simulink model "RLC"  (Simulink 7.5)
settings: Solver=ode3  StartTime=0.0  StopTime=4  FixedStep=1/32000  RelTol=1e-3
InitFcn:
  | RLC_datastruct
StopFcn:
  | PostProcessing
values from neighbouring files (symbols this model uses):
  CValue = 0.00068    [RLC_datastruct.m]
  LValue = 0.001    [RLC_datastruct.m]
  RValue = 2    [RLC_datastruct.m]
libraries: dspsrcs4 x1
settings Model: Creator=Zsolt  LastModifiedBy=bapty

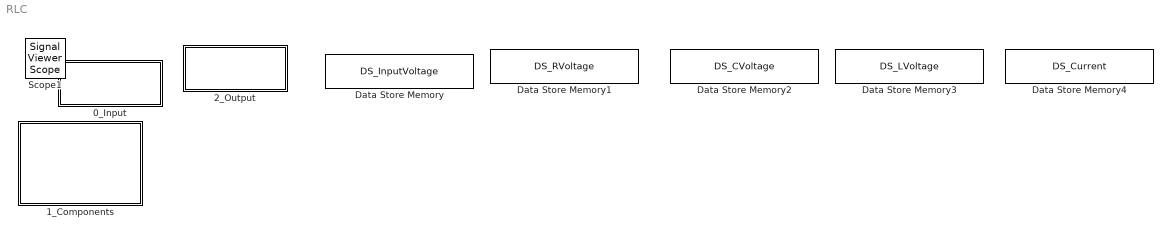
== system RLC ==
  0_Input : Subsystem
  1_Components : Subsystem
  2_Output : Subsystem
  Data Store Memory : DataStoreMemory  DataStoreName=DS_InputVoltage
  Data Store Memory1 : DataStoreMemory  DataStoreName=DS_RVoltage  ReadBeforeWriteMsg=warning  WriteAfterWriteMsg=warning  WriteAfterReadMsg=warning
  Data Store Memory2 : DataStoreMemory  DataStoreName=DS_CVoltage  ReadBeforeWriteMsg=warning  WriteAfterWriteMsg=warning  WriteAfterReadMsg=warning
  Data Store Memory3 : DataStoreMemory  DataStoreName=DS_LVoltage  ReadBeforeWriteMsg=warning  WriteAfterWriteMsg=warning  WriteAfterReadMsg=warning
  Data Store Memory4 : DataStoreMemory  DataStoreName=DS_Current  ReadBeforeWriteMsg=warning  WriteAfterWriteMsg=warning  WriteAfterReadMsg=warning
  Scope1 : SignalViewerScope  IOType=viewer  RefreshTime=0.035000

== system RLC/0_Input ==
  0_Chirp : dspsrcs4/Chirp  sweep=Linear  mode=Unidirectional  f0=1  f1=1000  t1=4  Tsweep=4  phase=0  Ts=1/32000  spf=1  datatype=Double
  1_Data Store Write : DataStoreWrite  DataStoreName=DS_InputVoltage  SampleTime=-1
  2_To Workspace : ToWorkspace  VariableName=InputVoltage  SampleTime=-1  SaveFormat=Structure With Time
  wires:
  0_Chirp/1 -> 1_Data Store Write/1, 2_To Workspace/1

== system RLC/1_Components ==
  RLC : Subsystem

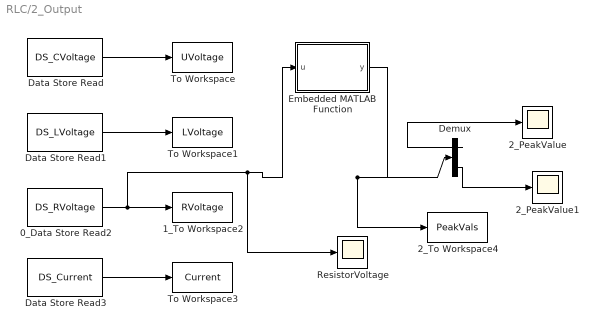
== system RLC/2_Output ==
  0_Data Store Read2 : DataStoreRead  DataStoreName=DS_RVoltage  SampleTime=-1
  1_To Workspace2 : ToWorkspace  VariableName=RVoltage  SampleTime=-1  SaveFormat=Structure With Time
  2_PeakValue : Scope
      settings: TimeRange=4  YMin=0  YMax=300  Decimation=10
  2_PeakValue1 : Scope
      settings: YMin=0  YMax=100  SaveName=ScopeData3  Decimation=10
  2_To Workspace4 : ToWorkspace  VariableName=PeakVals  SampleTime=-1  SaveFormat=Structure With Time
  Data Store Read : DataStoreRead  DataStoreName=DS_CVoltage  SampleTime=-1
  Data Store Read1 : DataStoreRead  DataStoreName=DS_LVoltage  SampleTime=-1
  Data Store Read3 : DataStoreRead  DataStoreName=DS_Current  SampleTime=-1
  Demux : Demux  Outputs=2
  Embedded MATLAB Function : Stateflow chart  TreatAsAtomicUnit=on
  ResistorVoltage : Scope
      settings: YMin=-1  YMax=1  SaveName=ScopeData2  Decimation=10
  To Workspace : ToWorkspace  VariableName=UVoltage  SampleTime=-1  SaveFormat=Structure With Time
  To Workspace1 : ToWorkspace  VariableName=LVoltage  SampleTime=-1  SaveFormat=Structure With Time
  To Workspace3 : ToWorkspace  VariableName=Current  SampleTime=-1  SaveFormat=Structure With Time
  wires:
  Data Store Read/1 -> To Workspace/1
  Data Store Read1/1 -> To Workspace1/1
  0_Data Store Read2/1 -> 1_To Workspace2/1, ResistorVoltage/1, Embedded MATLAB Function/1(u)
  Data Store Read3/1 -> To Workspace3/1
  Embedded MATLAB Function/1(y) -> Demux/1, 2_To Workspace4/1
  Demux/1 -> 2_PeakValue/1
  Demux/2 -> 2_PeakValue1/1

== system RLC/1_Components/RLC ==
  BondGraphDynamics : Subsystem
  Data Store Read : DataStoreRead  DataStoreName=DS_InputVoltage  SampleTime=-1
  wires:
  Data Store Read/1 -> BondGraphDynamics/1(InputVoltage)

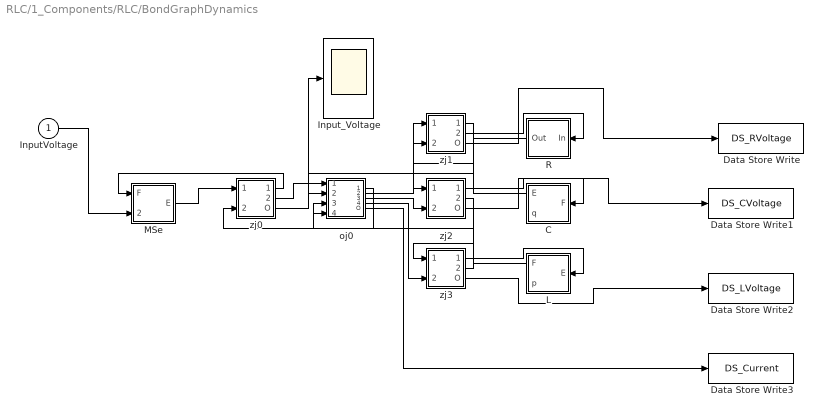
== system RLC/1_Components/RLC/BondGraphDynamics ==
  InputVoltage : Inport
  C : Subsystem  mask{C=CValue, IC=0}
      mask prompts: C "Value of C:"; IC "Initial Condition:"
      mask Display: image(imread('C.png','BackgroundColor',[1 1 1]))
  Data Store Write : DataStoreWrite  DataStoreName=DS_RVoltage  SampleTime=-1
  Data Store Write1 : DataStoreWrite  DataStoreName=DS_CVoltage  SampleTime=-1
  Data Store Write2 : DataStoreWrite  DataStoreName=DS_LVoltage  SampleTime=-1
  Data Store Write3 : DataStoreWrite  DataStoreName=DS_Current  SampleTime=-1
  Input_Voltage : Scope
  L : Subsystem  mask{I=LValue, IC=0}
      mask prompts: I "Value of I:"; IC "Initial Condition:"
      mask Display: image(imread('I.png','BackgroundColor',[1 1 1]))
  MSe : Subsystem
      mask Display: image(imread('MSe.png','BackgroundColor',[1 1 1]))
  R : Subsystem  mask{R=RValue}
      mask prompts: R "Value of R:"
      mask Display: image(imread('R.png','BackgroundColor',[1 1 1]))
  oj0 : Subsystem
      mask Display: image(imread('1.png','BackgroundColor',[1 1 1]))
  zj0 : Subsystem
      mask Display: image(imread('0.png','BackgroundColor',[1 1 1]))
  zj1 : Subsystem
      mask Display: image(imread('0.png','BackgroundColor',[1 1 1]))
  zj2 : Subsystem
      mask Display: image(imread('0.png','BackgroundColor',[1 1 1]))
  zj3 : Subsystem
      mask Display: image(imread('0.png','BackgroundColor',[1 1 1]))
  wires:
  MSe/1(E) -> zj0/1(u(1))
  zj0/1(y(1)) -> MSe/1(F)
  zj0/2(y(2)) -> oj0/1(u(1))
  oj0/1(y(1)) -> zj0/2(u(2))
  oj0/2(y(2)) -> zj1/1(u(1))
  zj1/1(y(1)) -> oj0/2(u(2))
  oj0/3(y(3)) -> zj2/2(u(2))
  zj2/2(y(2)) -> oj0/3(u(3))
  oj0/4(y(4)) -> zj3/2(u(2))
  zj3/2(y(2)) -> oj0/4(u(4))
  zj1/2(y(2)) -> R/1(In)
  R/1(Out) -> zj1/2(u(2))
  zj2/1(y(1)) -> C/1(F)
  C/1(E) -> zj2/1(u(1))
  zj3/1(y(1)) -> L/1(E)
  L/1(F) -> zj3/1(u(1))
  InputVoltage/1 -> MSe/2(Se Value)
  zj3/3(O) -> Data Store Write2/1
  zj2/3(O) -> Data Store Write1/1
  zj1/3(O) -> Data Store Write/1
  zj0/3(O) -> Input_Voltage/1
  oj0/5(O) -> Data Store Write3/1

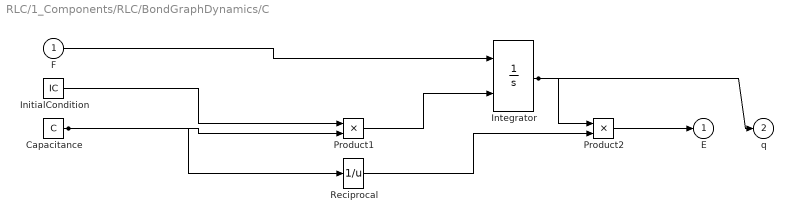
== system RLC/1_Components/RLC/BondGraphDynamics/C ==
  F : Inport
  Capacitance : Constant  Value=C
  InitialCondition : Constant  Value=IC
  Integrator : Integrator  InitialConditionSource=external
  Product1 : Product  SaturateOnIntegerOverflow=on  RndMeth=Zero  InputSameDT=on  OutDataTypeStr=Inherit: Same as first input
  Product2 : Product  SaturateOnIntegerOverflow=on  RndMeth=Zero  InputSameDT=on  OutDataTypeStr=Inherit: Same as first input
  Reciprocal : Math  Operator=reciprocal  SaturateOnIntegerOverflow=on
  E : Outport
  q : Outport  Port=2
  wires:
  F/1 -> Integrator/1
  InitialCondition/1 -> Product1/1
  Capacitance/1 -> Reciprocal/1, Product1/2
  Product1/1 -> Integrator/2
  Integrator/1 -> Product2/1, q/1
  Reciprocal/1 -> Product2/2
  Product2/1 -> E/1

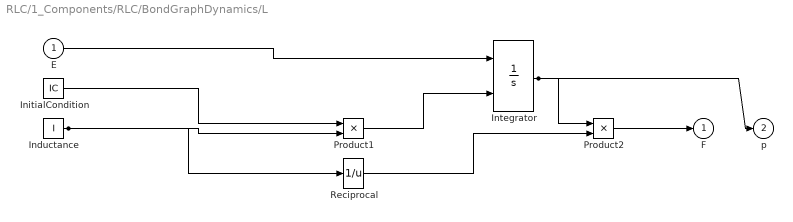
== system RLC/1_Components/RLC/BondGraphDynamics/L ==
  E : Inport
  Inductance : Constant  Value=I
  InitialCondition : Constant  Value=IC
  Integrator : Integrator  InitialConditionSource=external
  Product1 : Product  SaturateOnIntegerOverflow=on  RndMeth=Zero  InputSameDT=on  OutDataTypeStr=Inherit: Same as first input
  Product2 : Product  SaturateOnIntegerOverflow=on  RndMeth=Zero  InputSameDT=on  OutDataTypeStr=Inherit: Same as first input
  Reciprocal : Math  Operator=reciprocal  SaturateOnIntegerOverflow=on
  F : Outport
  p : Outport  Port=2
  wires:
  E/1 -> Integrator/1
  InitialCondition/1 -> Product1/1
  Inductance/1 -> Reciprocal/1, Product1/2
  Product1/1 -> Integrator/2
  Integrator/1 -> Product2/1, p/1
  Reciprocal/1 -> Product2/2
  Product2/1 -> F/1

== system RLC/1_Components/RLC/BondGraphDynamics/MSe ==
  F : Inport
  Se Value : Inport  Port=2
  E : Outport
  wires:
  Se Value/1 -> E/1

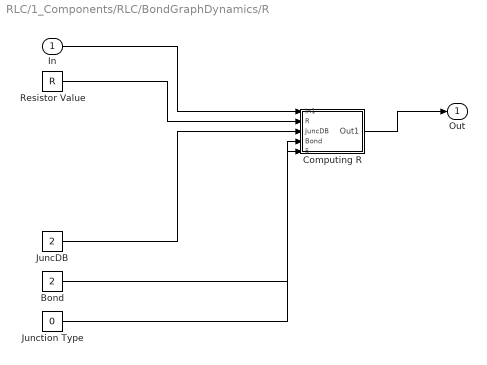
== system RLC/1_Components/RLC/BondGraphDynamics/R ==
  In : Inport
  Bond : Constant  Value=2
  Computing R : Subsystem
  JuncDB : Constant  Value=2
  Junction Type : Constant  Value=0
  Resistor Value : Constant  Value=R
  Out : Outport
  wires:
  In/1 -> Computing R/1(In1)
  Resistor Value/1 -> Computing R/2(R)
  JuncDB/1 -> Computing R/3(JuncDB)
  Bond/1 -> Computing R/4(Bond)
  Junction Type/1 -> Computing R/5(Junction Type)
  Computing R/1(Out1) -> Out/1

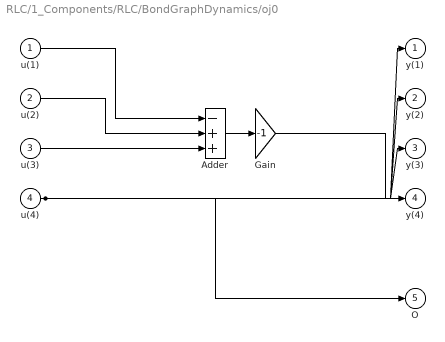
== system RLC/1_Components/RLC/BondGraphDynamics/oj0 ==
  u(1) : Inport
  u(2) : Inport  Port=2
  u(3) : Inport  Port=3
  u(4) : Inport  Port=4
  Adder : Sum  Inputs=-++  SaturateOnIntegerOverflow=on  InputSameDT=on  OutDataTypeStr=Inherit: Same as first input
  Gain : Gain  Gain=-1  SaturateOnIntegerOverflow=on  OutDataTypeStr=Inherit: Same as input  ParamDataTypeStr=Inherit: Same as input
  y(1) : Outport
  y(2) : Outport  Port=2
  y(3) : Outport  Port=3
  y(4) : Outport  Port=4
  O : Outport  Port=5
  wires:
  Adder/1 -> Gain/1
  u(4)/1 -> y(1)/1, y(2)/1, y(3)/1, O/1
  u(1)/1 -> Adder/1
  u(2)/1 -> Adder/2
  u(3)/1 -> Adder/3
  Gain/1 -> y(4)/1

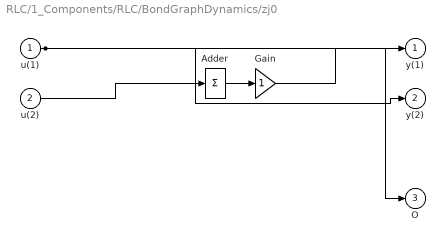
== system RLC/1_Components/RLC/BondGraphDynamics/zj0 ==
  u(1) : Inport
  u(2) : Inport  Port=2
  Adder : Sum  Inputs=+  SaturateOnIntegerOverflow=on  InputSameDT=on  OutDataTypeStr=Inherit: Same as first input
  Gain : Gain  SaturateOnIntegerOverflow=on  OutDataTypeStr=Inherit: Same as input  ParamDataTypeStr=Inherit: Same as input
  y(1) : Outport
  y(2) : Outport  Port=2
  O : Outport  Port=3
  wires:
  Adder/1 -> Gain/1
  Gain/1 -> y(1)/1
  u(1)/1 -> y(2)/1, O/1
  u(2)/1 -> Adder/1

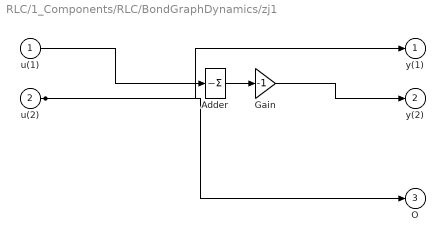
== system RLC/1_Components/RLC/BondGraphDynamics/zj1 ==
  u(1) : Inport
  u(2) : Inport  Port=2
  Adder : Sum  Inputs=-  SaturateOnIntegerOverflow=on  InputSameDT=on  OutDataTypeStr=Inherit: Same as first input
  Gain : Gain  Gain=-1  SaturateOnIntegerOverflow=on  OutDataTypeStr=Inherit: Same as input  ParamDataTypeStr=Inherit: Same as input
  y(1) : Outport
  y(2) : Outport  Port=2
  O : Outport  Port=3
  wires:
  Adder/1 -> Gain/1
  u(2)/1 -> y(1)/1, O/1
  u(1)/1 -> Adder/1
  Gain/1 -> y(2)/1

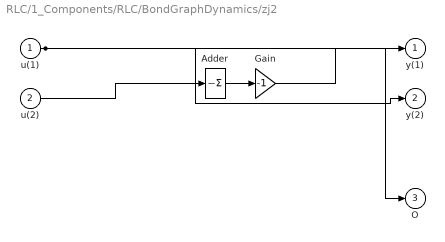
== system RLC/1_Components/RLC/BondGraphDynamics/zj2 ==
  u(1) : Inport
  u(2) : Inport  Port=2
  Adder : Sum  Inputs=-  SaturateOnIntegerOverflow=on  InputSameDT=on  OutDataTypeStr=Inherit: Same as first input
  Gain : Gain  Gain=-1  SaturateOnIntegerOverflow=on  OutDataTypeStr=Inherit: Same as input  ParamDataTypeStr=Inherit: Same as input
  y(1) : Outport
  y(2) : Outport  Port=2
  O : Outport  Port=3
  wires:
  Adder/1 -> Gain/1
  Gain/1 -> y(1)/1
  u(1)/1 -> y(2)/1, O/1
  u(2)/1 -> Adder/1

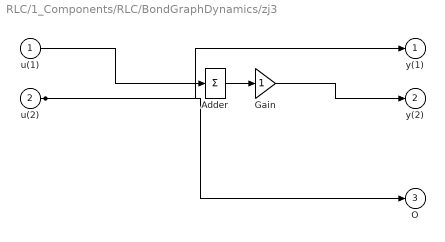
== system RLC/1_Components/RLC/BondGraphDynamics/zj3 ==
  u(1) : Inport
  u(2) : Inport  Port=2
  Adder : Sum  Inputs=+  SaturateOnIntegerOverflow=on  InputSameDT=on  OutDataTypeStr=Inherit: Same as first input
  Gain : Gain  SaturateOnIntegerOverflow=on  OutDataTypeStr=Inherit: Same as input  ParamDataTypeStr=Inherit: Same as input
  y(1) : Outport
  y(2) : Outport  Port=2
  O : Outport  Port=3
  wires:
  Adder/1 -> Gain/1
  u(2)/1 -> y(1)/1, O/1
  u(1)/1 -> Adder/1
  Gain/1 -> y(2)/1

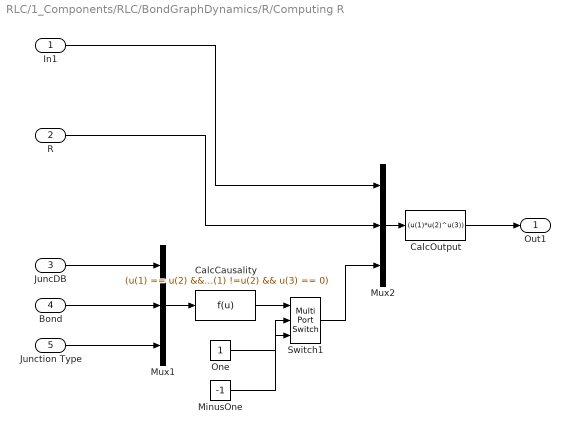
== system RLC/1_Components/RLC/BondGraphDynamics/R/Computing R ==
  In1 : Inport
  R : Inport  Port=2
  JuncDB : Inport  Port=3
  Bond : Inport  Port=4
  Junction Type : Inport  Port=5
  CalcCausality : Fcn  Expr=(u(1) == u(2) && u(3) ==1) || (u(1) !=u(2) && u(3) == 0)
  CalcOutput : Fcn  Expr=(u(1)*u(2)^u(3))
  MinusOne : Constant  Value=-1
  Mux1 : Mux  Inputs=3
  Mux2 : Mux  Inputs=3
  One : Constant
  Switch1 : MultiPortSwitch  DataPortOrder=Zero-based contiguous  Inputs=2  zeroidx=on  SaturateOnIntegerOverflow=on  InputSameDT=on
  Out1 : Outport
  wires:
  In1/1 -> Mux2/1
  R/1 -> Mux2/2
  JuncDB/1 -> Mux1/1
  Bond/1 -> Mux1/2
  Junction Type/1 -> Mux1/3
  Mux1/1 -> CalcCausality/1
  CalcCausality/1 -> Switch1/1
  One/1 -> Switch1/2
  MinusOne/1 -> Switch1/3
  Switch1/1 -> Mux2/3
  Mux2/1 -> CalcOutput/1
  CalcOutput/1 -> Out1/1

== matlab function 2_Output/Embedded MATLAB Function ==
  data: u input double; y output double
function y = fcn(u)
%#eml
persistent prevDat;
persistent wind;
if isempty(prevDat)
  prevDat = zeros(1,1024);
  wind = hamming(1024)';
end
tmpDat = [prevDat u];
prevDat = tmpDat(2:length(tmpDat));
fhist = abs(fft(prevDat.*wind));
%fhist = abs(fft(prevDat));
[val idx] = max(fhist);
if val > 1000 
  val = 0;
 end
 result = [val idx];

y = result;
